simulink model "test_newfft"  (Simulink 6.2)
settings: Solver=ode45  StartTime=0.0  StopTime=100  RelTol=1e-3
libraries: xbsIndex_r3 x265, simulink x1
(part 2 of 4)

== system test_newfft/r2_dit_fft/r2_dit_stage_1 ==
  a_in : Inport  Port=1  LatchInput=off
  b_in : Inport  Port=2  LatchInput=off
  sync_in : Inport  Port=3  LatchInput=off
  biplex_commutator : Subsystem  mask(Biplex Commutator){log2_size=4, n_bits=8, use_bram=off}
      mask prompts: log2_size "Log2 Block Size"; n_bits "Bit Width"; use_bram "Use BRAM"
      mask help: The biplex commutator commutes the first half of the BloBhi input "block" with the last half of the AloAhi input "block". A "block" is 2^log2_size consecutive samples (i.e. always a power of 2). sync_in precedes the first data input sample by one clock cycle. Overall latency from sync_in to sync_out is 2^(log2_size-1)+1.
      settings: AttributesFormatString=|
      | size = 16
      | delay slr
      mask Help:
      | <pre>
      | Description::
      | 
      | The biplex commutator commutes the first half of the BloBhi input "block"  with the last half
      | of the AloAhi input "block".  A "block" is 2^log2_size consecutive samples (i.e. always a
      | power of 2).
      | 
      | sync_in precedes the first data input sample by one clock cycle.
      | sync_out precedes the corresponding output sample by one clock cycle.
      | Overall latency from sync_in to sync_out is 2^(N-1)+1.
      | 
      | Mask Parameters::
      | 
      | Log 2 Block Size (log2_size): The base-2 logarithm of the length of one complete input block.
      | This MUST be an integer because the current implementation requires that
      | the input block size MUST be a power of 2.  (aka "N")
      | 
      | Bit Width (n_bits): Specifies the width of the real/imaginary components.
      | Width of each component is assumed equal.
      | 
      | Use BRAM (use_bram): Check this checkbox to implement the internal delays using BRAM.
      | If unchecked, the internal delays will be implemented using SLR16 elements.
      | </pre>
  r2_butterfly : Subsystem  mask(Radix-2 Butterfly){n_bits=8, shift=0, quantization=Truncate, add_latency=1}
      mask prompts: n_bits "Bit Width In"; shift "Shift Bits"; add_latency "Adder Latency"
      mask help: The radix-2 butterfly produces a+b and a-b outputs for a and b inputs.
      settings: AttributesFormatString=shift 0
      mask Help:
      | <pre>
      | Description::
      | 
      | The radix-2 butterfly produces a+b and a-b outputs for a and b inputs.
      | The outputs are one bit wider than the inputs.
      | The output precision (i.e. the number of fractional bits) stays the same.
      | 
      | Mask Parameters::
      | 
      | Bit Width In (n_bits): Specifies the width of the real/imaginary components.
      | Width of each component is assumed equal.
      | 
      | Shift Bits (shift): Specifies how many bits to shift (down) by.  A positive value causes
      | the specified number of least significant bits to be dropped.  Usually zero or positive values
      | are used to permit or limit bit growth, but negative values can be used to induce bit growth.
      | 
      | Quantization (quantization): Specifies quantization handling (when shift bits > 0).
      | 
      | Adder Latency (add_latency): Latency to use for the underlying real adders.
      | </pre>
      mask StyleString: edit,edit,popup(Truncate|Round  (unbiased: +/- Inf)|Round  (unbiased: Even Values)),edit
  r2_twiddle : Subsystem
      mask Type: Radix-2 Stage-1 Twiddle Stage
      mask Description: A stage-1 twiddle stage for radix-2 Fast Fourier Transforms. Since there are no twiddles in stage 1 of an FFT, this is just a dummy placeholder block that passes its inputs through to its outputs.    Since it is a no-op, its use is completely optional.
      mask Help:
      | <pre>
      | Description::
      | 
      | A stage-1 twiddle stage for radix-2 Fast Fourier Transforms.
      | 
      | Since there are no twiddles in stage 1 of an FFT, this is just a dummy placeholder
      | block that passes its inputs through to its outputs.
      | 
      | Since it is a no-op, its use is completely optional.
      | 
      | Note that stages are counted from 1 to n_stages for DIT (i.e. cur_stage==1 for the first stage)
      | and n_stages to 1for DIF (i.e. cur_stage==1 for the last stage).  Therefore, this block, if used,
      | should be the first twiddle stage of a DIT FFT or the last twiddle stage of a DIF FFT.
      | 
      | Mask Parameters::
      | 
      | (N/A)
  a_out : Outport
  b_out : Outport  Port=2
  sync_out : Outport  Port=3
  wires:
  r2_butterfly/3(sync_out) -> sync_out/1
  r2_butterfly/2(a-b) -> b_out/1
  r2_butterfly/1(a+b) -> a_out/1
  sync_in/1 -> biplex_commutator/3(sync_in)
  b_in/1 -> biplex_commutator/2(BloBhi)
  a_in/1 -> biplex_commutator/1(AloAhi)
  biplex_commutator/3(sync_out) -> r2_twiddle/3(sync_in)
  biplex_commutator/2(AhiBhi) -> r2_twiddle/2(b_in)
  biplex_commutator/1(AloBlo) -> r2_twiddle/1(a_in)
  r2_twiddle/1(a_out) -> r2_butterfly/1(a)
  r2_twiddle/2(b_out) -> r2_butterfly/2(b)
  r2_twiddle/3(sync_out) -> r2_butterfly/3(sync_in)

== system test_newfft/r2_dit_fft/r2_dit_stage_2 ==
  a_in : Inport  Port=1  LatchInput=off
  b_in : Inport  Port=2  LatchInput=off
  sync_in : Inport  Port=3  LatchInput=off
  biplex_commutator : Subsystem  mask(Biplex Commutator){log2_size=3, n_bits=9, use_bram=off}
      mask prompts: log2_size "Log2 Block Size"; n_bits "Bit Width"; use_bram "Use BRAM"
      mask help: The biplex commutator commutes the first half of the BloBhi input "block" with the last half of the AloAhi input "block". A "block" is 2^log2_size consecutive samples (i.e. always a power of 2). sync_in precedes the first data input sample by one clock cycle. Overall latency from sync_in to sync_out is 2^(log2_size-1)+1.
      settings: AttributesFormatString=|
      | size = 8
      | delay slr
      mask Help:
      | <pre>
      | Description::
      | 
      | The biplex commutator commutes the first half of the BloBhi input "block"  with the last half
      | of the AloAhi input "block".  A "block" is 2^log2_size consecutive samples (i.e. always a
      | power of 2).
      | 
      | sync_in precedes the first data input sample by one clock cycle.
      | sync_out precedes the corresponding output sample by one clock cycle.
      | Overall latency from sync_in to sync_out is 2^(N-1)+1.
      | 
      | Mask Parameters::
      | 
      | Log 2 Block Size (log2_size): The base-2 logarithm of the length of one complete input block.
      | This MUST be an integer because the current implementation requires that
      | the input block size MUST be a power of 2.  (aka "N")
      | 
      | Bit Width (n_bits): Specifies the width of the real/imaginary components.
      | Width of each component is assumed equal.
      | 
      | Use BRAM (use_bram): Check this checkbox to implement the internal delays using BRAM.
      | If unchecked, the internal delays will be implemented using SLR16 elements.
      | </pre>
  r2_butterfly : Subsystem  mask(Radix-2 Butterfly with optional -j twiddle (DIT, twiddle before butterfly)){n_bits=9, shift=0, quantization=Truncate, add_latency=1}
      mask prompts: n_bits "Bit Width In"; shift "Shift Bits"; add_latency "Adder Latency"
      mask help: The radix-2 butterfly produces a+b and a-b outputs for a and b inputs. This variation efficiently includes an optional -j twiddle factor that can be applied before the butterfly (suitable for use in stage two of a DIT FFT).
      settings: AttributesFormatString=shift 0
      mask Help:
      | <pre>
      | Description::
      | 
      | The radix-2 butterfly produces a+b and a-b outputs for a and b inputs.
      | This variation efficiently includes an optional -j twiddle factor that can be
      | applied before the butterfly (suitable for use in stage two of a DIT FFT).
      | 
      | The -j twiddle factor is applied to tbe b input when tw_en is high,
      | thus producing a-jb on the a+b output and a+jb on the a-b output.
      | 
      | The outputs are one bit wider than the inputs.
      | The output precision (i.e. the number of fractional bits) stays the same.
      | 
      | Mask Parameters::
      | 
      | Bit Width In (n_bits): Specifies the width of the real/imaginary components.
      | Width of each component is assumed equal.
      | 
      | Shift Bits (shift): Specifies how many bits to shift (down) by.  A positive value causes
      | the specified number of least significant bits to be dropped.  Usually zero or positive values
      | are used to permit or limit bit growth, but negative values can be used to induce bit growth.
      | 
      | Quantization (quantization): Specifies quantization handling (when shift bits > 0).
      | 
      | Adder Latency (add_latency): Latency to use for the underlying real adders.
      | </pre>
      mask StyleString: edit,edit,popup(Truncate|Round  (unbiased: +/- Inf)|Round  (unbiased: Even Values)),edit
  r2_twiddle : Subsystem  mask(Radix-2 DIT Stage-2 Twiddle Stage){n_stages=4}
      mask prompts: n_stages "Total Stages"
      mask help: A stage-2 twiddle stage for radix-2 Decimation in Time Fast Fourier Transforms. The FFT is assumed to have inputs in normal order and outputs in bit-reversed order. This block must be used in conjuction with an r2_butterfly_dit_j_opt block (or equivalent) which has an optional -j twiddle factor built in.
      mask Help:
      | <pre>
      | Description::
      | 
      | A stage-2 twiddle stage for radix-2 Decimation in Time Fast Fourier Transforms.
      | 
      | The FFT is assumed to have inputs in normal order and outputs in bit-reversed order.
      | 
      | This block must be used in conjuction with an r2_butterfly_dit_j_opt block (or equivalent)
      | which has an optional -j twiddle factor built in.  This block does no twidlling at all; it just provides
      | a tw_en output for use with an r2_butterfly_dit_j_opt block (or equivalent).
      | 
      | Mask Parameters::
      | 
      | Total Stages (n_stages):  The number of total stages in the FFT.
      | The FFT will have 2^n_stages points.
  a_out : Outport
  b_out : Outport  Port=2
  sync_out : Outport  Port=3
  wires:
  r2_butterfly/3(sync_out) -> sync_out/1
  r2_butterfly/2(a-b) -> b_out/1
  r2_butterfly/1(a+b) -> a_out/1
  sync_in/1 -> biplex_commutator/3(sync_in)
  b_in/1 -> biplex_commutator/2(BloBhi)
  a_in/1 -> biplex_commutator/1(AloAhi)
  biplex_commutator/3(sync_out) -> r2_twiddle/3(sync_in)
  biplex_commutator/2(AhiBhi) -> r2_twiddle/2(b_in)
  biplex_commutator/1(AloBlo) -> r2_twiddle/1(a_in)
  r2_twiddle/1(a_out) -> r2_butterfly/1(a)
  r2_twiddle/2(b_out) -> r2_butterfly/2(b)
  r2_twiddle/3(sync_out) -> r2_butterfly/3(sync_in)
  r2_twiddle/4(tw_en) -> r2_butterfly/4(tw_en)

== system test_newfft/r2_dit_fft/r2_dit_stage_3 ==
  a_in : Inport  Port=1  LatchInput=off
  b_in : Inport  Port=2  LatchInput=off
  sync_in : Inport  Port=3  LatchInput=off
  biplex_commutator : Subsystem  mask(Biplex Commutator){log2_size=2, n_bits=10, use_bram=off}
      mask prompts: log2_size "Log2 Block Size"; n_bits "Bit Width"; use_bram "Use BRAM"
      mask help: The biplex commutator commutes the first half of the BloBhi input "block" with the last half of the AloAhi input "block". A "block" is 2^log2_size consecutive samples (i.e. always a power of 2). sync_in precedes the first data input sample by one clock cycle. Overall latency from sync_in to sync_out is 2^(log2_size-1)+1.
      settings: AttributesFormatString=|
      | size = 4
      | delay slr
      mask Help:
      | <pre>
      | Description::
      | 
      | The biplex commutator commutes the first half of the BloBhi input "block"  with the last half
      | of the AloAhi input "block".  A "block" is 2^log2_size consecutive samples (i.e. always a
      | power of 2).
      | 
      | sync_in precedes the first data input sample by one clock cycle.
      | sync_out precedes the corresponding output sample by one clock cycle.
      | Overall latency from sync_in to sync_out is 2^(N-1)+1.
      | 
      | Mask Parameters::
      | 
      | Log 2 Block Size (log2_size): The base-2 logarithm of the length of one complete input block.
      | This MUST be an integer because the current implementation requires that
      | the input block size MUST be a power of 2.  (aka "N")
      | 
      | Bit Width (n_bits): Specifies the width of the real/imaginary components.
      | Width of each component is assumed equal.
      | 
      | Use BRAM (use_bram): Check this checkbox to implement the internal delays using BRAM.
      | If unchecked, the internal delays will be implemented using SLR16 elements.
      | </pre>
  r2_butterfly : Subsystem  mask(Radix-2 Butterfly){n_bits=10, shift=0, quantization=Truncate, add_latency=1}
      mask prompts: n_bits "Bit Width In"; shift "Shift Bits"; add_latency "Adder Latency"
      mask help: The radix-2 butterfly produces a+b and a-b outputs for a and b inputs.
      settings: AttributesFormatString=shift 0
      mask Help:
      | <pre>
      | Description::
      | 
      | The radix-2 butterfly produces a+b and a-b outputs for a and b inputs.
      | The outputs are one bit wider than the inputs.
      | The output precision (i.e. the number of fractional bits) stays the same.
      | 
      | Mask Parameters::
      | 
      | Bit Width In (n_bits): Specifies the width of the real/imaginary components.
      | Width of each component is assumed equal.
      | 
      | Shift Bits (shift): Specifies how many bits to shift (down) by.  A positive value causes
      | the specified number of least significant bits to be dropped.  Usually zero or positive values
      | are used to permit or limit bit growth, but negative values can be used to induce bit growth.
      | 
      | Quantization (quantization): Specifies quantization handling (when shift bits > 0).
      | 
      | Adder Latency (add_latency): Latency to use for the underlying real adders.
      | </pre>
      mask StyleString: edit,edit,popup(Truncate|Round  (unbiased: +/- Inf)|Round  (unbiased: Even Values)),edit
  r2_twiddle : Subsystem  mask(Radix-2 General Twiddle Stage){n_stages=4, cur_stage=3, decimation=Time, n_bits=10, bin_pt=7, n_bits_w=9, use_bram=off, mult_latency=3, add_latency=1}
      mask prompts: n_stages "Total Stages"; cur_stage "Current Stage"; decimation "Decimation Mode"; n_bits "Number of Bits In/Out"; bin_pt "Binary Point In/Out"; n_bits_w "Twiddle Coefficient Bitwidth"; use_bram "Use BRAM For Twiddle Coefficients"; mult_latency "Multiplier Latency"; add_latency "Adder Latency"
      mask help: A general twiddle stage for radix-2 Fast Fourier Transforms. Can be used in Decimation in Time (i.e. twiddles before butterflies) or Decimation in Frequency (i.e. twiddles after butterflies) FFTs. Regardless of the decimation mode, the FFT is assumed to have inputs in normal order and outputs in bit-reversed order.
      settings: AttributesFormatString=4 twiddles in dist
      mask Help:
      | <pre>
      | Description::
      | 
      | A general twiddle stage for radix-2 Fast Fourier Transforms.
      | 
      | Can be used in  Decimation in Time (i.e. twiddles before butterflies) or Decimation in Frequency
      | (i.e. twiddles after butterflies) FFTs.  Regardless of the decimation mode, the FFT is assumed
      | to have inputs in normal order and outputs in bit-reversed order.
      | 
      | Input a_in is passed through unchanged to a_out, while input b is passed through to bw after
      | being "twiddled".  Since twiddling is effectively multiplication by a complex number with unity
      | magnitude, the bit respresentation of bw is the same as b (i.e. twiddling does not cause bit
      | growth).  Input a_in is assumed to have the same bit width as b.  Thus, a_in, a_out, b, and
      | bw all have the same bit representation.
      | 
      | Mask Parameters::
      | 
      | Total Stages (n_stages):  The number of total stages in the FFT.
      | The FFT will have 2^n_stages points.
      | 
      | Current Stage (cur_stage):  The number of the current stage for which this block should
      | generate twiddle coefficients.  Valid values are 3 through n_stages, inclusive.  Note that
      | stages are counted from 1 to n_stages for DIT (i.e. cur_stage==1 for the first stage) and
      | n_stages to 1 for DIF (i.e. cur_stage==1 for the last stage).
      | 
      | Decimation Mode (decimation): The decimation mode of the FFT.
      | 
      | Number of Bits In/Out (n_bits): Specifies the width of the real/imaginary
      | components of ports a_in, b, a_out, bw.  Assumed equal for both components.
      | 
      | Binary Point In/Out (bin_pt): Specifies the binary point position of the real/imaginary
      | components of ports a_in, b, a_out, bw.  Assumed equal for both components.
      | 
      | Twiddle Coefficient Bitwidth (n_bits_w): Specifies the width of the real/imaginary
      | components of the twiddle coefficients.  Assumed equal for both components.
      | 
      | Use BRAM for Twiddle Coefficients (use_bram): Check this checkbox to store twiddle
      | coefficients in BRAM.  If unchecked, the twiddle coefficients will be sored in distributed
      | memory (i.e. slices).
      | 
      | Multiplier Latency (mult_latency): Latency to use for the underlying real multipliers.
      | 
      | Adder Latency (add_latency): Latency to use for the underlying real adders.
      mask StyleString: edit,edit,popup(Time|Frequency),edit,edit,edit,checkbox,edit,edit
  a_out : Outport
  b_out : Outport  Port=2
  sync_out : Outport  Port=3
  wires:
  r2_butterfly/3(sync_out) -> sync_out/1
  r2_butterfly/2(a-b) -> b_out/1
  r2_butterfly/1(a+b) -> a_out/1
  sync_in/1 -> biplex_commutator/3(sync_in)
  b_in/1 -> biplex_commutator/2(BloBhi)
  a_in/1 -> biplex_commutator/1(AloAhi)
  biplex_commutator/3(sync_out) -> r2_twiddle/3(sync_in)
  biplex_commutator/2(AhiBhi) -> r2_twiddle/2(b)
  biplex_commutator/1(AloBlo) -> r2_twiddle/1(a_in)
  r2_twiddle/1(a_out) -> r2_butterfly/1(a)
  r2_twiddle/2(bw) -> r2_butterfly/2(b)
  r2_twiddle/3(sync_out) -> r2_butterfly/3(sync_in)

== system test_newfft/r2_dit_fft/r2_dit_stage_4 ==
  a_in : Inport  Port=1  LatchInput=off
  b_in : Inport  Port=2  LatchInput=off
  sync_in : Inport  Port=3  LatchInput=off
  biplex_commutator : Subsystem  mask(Biplex Commutator){log2_size=1, n_bits=11, use_bram=off}
      mask prompts: log2_size "Log2 Block Size"; n_bits "Bit Width"; use_bram "Use BRAM"
      mask help: The biplex commutator commutes the first half of the BloBhi input "block" with the last half of the AloAhi input "block". A "block" is 2^log2_size consecutive samples (i.e. always a power of 2). sync_in precedes the first data input sample by one clock cycle. Overall latency from sync_in to sync_out is 2^(log2_size-1)+1.
      settings: AttributesFormatString=|
      | size = 2
      | delay slr
      mask Help:
      | <pre>
      | Description::
      | 
      | The biplex commutator commutes the first half of the BloBhi input "block"  with the last half
      | of the AloAhi input "block".  A "block" is 2^log2_size consecutive samples (i.e. always a
      | power of 2).
      | 
      | sync_in precedes the first data input sample by one clock cycle.
      | sync_out precedes the corresponding output sample by one clock cycle.
      | Overall latency from sync_in to sync_out is 2^(N-1)+1.
      | 
      | Mask Parameters::
      | 
      | Log 2 Block Size (log2_size): The base-2 logarithm of the length of one complete input block.
      | This MUST be an integer because the current implementation requires that
      | the input block size MUST be a power of 2.  (aka "N")
      | 
      | Bit Width (n_bits): Specifies the width of the real/imaginary components.
      | Width of each component is assumed equal.
      | 
      | Use BRAM (use_bram): Check this checkbox to implement the internal delays using BRAM.
      | If unchecked, the internal delays will be implemented using SLR16 elements.
      | </pre>
  r2_butterfly : Subsystem  mask(Radix-2 Butterfly){n_bits=11, shift=0, quantization=Truncate, add_latency=1}
      mask prompts: n_bits "Bit Width In"; shift "Shift Bits"; add_latency "Adder Latency"
      mask help: The radix-2 butterfly produces a+b and a-b outputs for a and b inputs.
      settings: AttributesFormatString=shift 0
      mask Help:
      | <pre>
      | Description::
      | 
      | The radix-2 butterfly produces a+b and a-b outputs for a and b inputs.
      | The outputs are one bit wider than the inputs.
      | The output precision (i.e. the number of fractional bits) stays the same.
      | 
      | Mask Parameters::
      | 
      | Bit Width In (n_bits): Specifies the width of the real/imaginary components.
      | Width of each component is assumed equal.
      | 
      | Shift Bits (shift): Specifies how many bits to shift (down) by.  A positive value causes
      | the specified number of least significant bits to be dropped.  Usually zero or positive values
      | are used to permit or limit bit growth, but negative values can be used to induce bit growth.
      | 
      | Quantization (quantization): Specifies quantization handling (when shift bits > 0).
      | 
      | Adder Latency (add_latency): Latency to use for the underlying real adders.
      | </pre>
      mask StyleString: edit,edit,popup(Truncate|Round  (unbiased: +/- Inf)|Round  (unbiased: Even Values)),edit
  r2_twiddle : Subsystem  mask(Radix-2 General Twiddle Stage){n_stages=4, cur_stage=4, decimation=Time, n_bits=11, bin_pt=7, n_bits_w=9, use_bram=off, mult_latency=3, add_latency=1}
      mask prompts: n_stages "Total Stages"; cur_stage "Current Stage"; decimation "Decimation Mode"; n_bits "Number of Bits In/Out"; bin_pt "Binary Point In/Out"; n_bits_w "Twiddle Coefficient Bitwidth"; use_bram "Use BRAM For Twiddle Coefficients"; mult_latency "Multiplier Latency"; add_latency "Adder Latency"
      mask help: A general twiddle stage for radix-2 Fast Fourier Transforms. Can be used in Decimation in Time (i.e. twiddles before butterflies) or Decimation in Frequency (i.e. twiddles after butterflies) FFTs. Regardless of the decimation mode, the FFT is assumed to have inputs in normal order and outputs in bit-reversed order.
      settings: AttributesFormatString=8 twiddles in dist
      mask Help:
      | <pre>
      | Description::
      | 
      | A general twiddle stage for radix-2 Fast Fourier Transforms.
      | 
      | Can be used in  Decimation in Time (i.e. twiddles before butterflies) or Decimation in Frequency
      | (i.e. twiddles after butterflies) FFTs.  Regardless of the decimation mode, the FFT is assumed
      | to have inputs in normal order and outputs in bit-reversed order.
      | 
      | Input a_in is passed through unchanged to a_out, while input b is passed through to bw after
      | being "twiddled".  Since twiddling is effectively multiplication by a complex number with unity
      | magnitude, the bit respresentation of bw is the same as b (i.e. twiddling does not cause bit
      | growth).  Input a_in is assumed to have the same bit width as b.  Thus, a_in, a_out, b, and
      | bw all have the same bit representation.
      | 
      | Mask Parameters::
      | 
      | Total Stages (n_stages):  The number of total stages in the FFT.
      | The FFT will have 2^n_stages points.
      | 
      | Current Stage (cur_stage):  The number of the current stage for which this block should
      | generate twiddle coefficients.  Valid values are 3 through n_stages, inclusive.  Note that
      | stages are counted from 1 to n_stages for DIT (i.e. cur_stage==1 for the first stage) and
      | n_stages to 1 for DIF (i.e. cur_stage==1 for the last stage).
      | 
      | Decimation Mode (decimation): The decimation mode of the FFT.
      | 
      | Number of Bits In/Out (n_bits): Specifies the width of the real/imaginary
      | components of ports a_in, b, a_out, bw.  Assumed equal for both components.
      | 
      | Binary Point In/Out (bin_pt): Specifies the binary point position of the real/imaginary
      | components of ports a_in, b, a_out, bw.  Assumed equal for both components.
      | 
      | Twiddle Coefficient Bitwidth (n_bits_w): Specifies the width of the real/imaginary
      | components of the twiddle coefficients.  Assumed equal for both components.
      | 
      | Use BRAM for Twiddle Coefficients (use_bram): Check this checkbox to store twiddle
      | coefficients in BRAM.  If unchecked, the twiddle coefficients will be sored in distributed
      | memory (i.e. slices).
      | 
      | Multiplier Latency (mult_latency): Latency to use for the underlying real multipliers.
      | 
      | Adder Latency (add_latency): Latency to use for the underlying real adders.
      mask StyleString: edit,edit,popup(Time|Frequency),edit,edit,edit,checkbox,edit,edit
  a_out : Outport
  b_out : Outport  Port=2
  sync_out : Outport  Port=3
  wires:
  r2_butterfly/3(sync_out) -> sync_out/1
  r2_butterfly/2(a-b) -> b_out/1
  r2_butterfly/1(a+b) -> a_out/1
  sync_in/1 -> biplex_commutator/3(sync_in)
  b_in/1 -> biplex_commutator/2(BloBhi)
  a_in/1 -> biplex_commutator/1(AloAhi)
  biplex_commutator/3(sync_out) -> r2_twiddle/3(sync_in)
  biplex_commutator/2(AhiBhi) -> r2_twiddle/2(b)
  biplex_commutator/1(AloBlo) -> r2_twiddle/1(a_in)
  r2_twiddle/1(a_out) -> r2_butterfly/1(a)
  r2_twiddle/2(bw) -> r2_butterfly/2(b)
  r2_twiddle/3(sync_out) -> r2_butterfly/3(sync_in)

== system test_newfft/r2_dit_fft/biplex_bitrev/bit_reverse ==
  in : Inport  Port=1  LatchInput=off
  bit0 : xbsIndex_r3/Slice  mode=Lower Bit Location + Width  nbits=1  bit1=0  base1=MSB of Input  bit0=0  base0=LSB of Input  boolean_output=off  explicit_period=off  period=1  dbl_ovrd=off
  bit1 : xbsIndex_r3/Slice  mode=Lower Bit Location + Width  nbits=1  bit1=0  base1=MSB of Input  bit0=1  base0=LSB of Input  boolean_output=off  explicit_period=off  period=1  dbl_ovrd=off
  bit2 : xbsIndex_r3/Slice  mode=Lower Bit Location + Width  nbits=1  bit1=0  base1=MSB of Input  bit0=2  base0=LSB of Input  boolean_output=off  explicit_period=off  period=1  dbl_ovrd=off
  concat : xbsIndex_r3/Concat  num_inputs=3  explicit_period=off  period=1  dbl_ovrd=off
  out : Outport
  wires:
  in/1 -> bit2/1, bit1/1, bit0/1
  bit2/1 -> concat/3
  bit1/1 -> concat/2
  bit0/1 -> concat/1
  concat/1 -> out/1

== system test_newfft/r2_dit_fft/biplex_bitrev/c_to_ri ==
  c : Inport  Port=1  LatchInput=off
  force_im : xbsIndex_r3/Reinterpret  force_arith_type=on  arith_type="Signed  (2's comp)"  force_bin_pt=on  bin_pt=0  force_valid=on
  force_re : xbsIndex_r3/Reinterpret  force_arith_type=on  arith_type="Signed  (2's comp)"  force_bin_pt=on  bin_pt=0  force_valid=on
  slice_im : xbsIndex_r3/Slice  mode=Lower Bit Location + Width  nbits=12  bit1=0  base1=MSB of Input  bit0=0  base0=LSB of Input  boolean_output=off  explicit_period=off  period=1  dbl_ovrd=off
  slice_re : xbsIndex_r3/Slice  mode=Upper Bit Location + Width  nbits=12  bit1=0  base1=MSB of Input  bit0=0  base0=LSB of Input  boolean_output=off  explicit_period=off  period=1  dbl_ovrd=off
  re : Outport
  im : Outport  Port=2
  wires:
  slice_re/1 -> force_re/1
  slice_im/1 -> force_im/1
  force_re/1 -> re/1
  force_im/1 -> im/1
  c/1 -> slice_re/1, slice_im/1

== system test_newfft/r2_dit_fft/biplex_bitrev/c_to_ri1 ==
  c : Inport  Port=1  LatchInput=off
  force_im : xbsIndex_r3/Reinterpret  force_arith_type=on  arith_type="Signed  (2's comp)"  force_bin_pt=on  bin_pt=0  force_valid=on
  force_re : xbsIndex_r3/Reinterpret  force_arith_type=on  arith_type="Signed  (2's comp)"  force_bin_pt=on  bin_pt=0  force_valid=on
  slice_im : xbsIndex_r3/Slice  mode=Lower Bit Location + Width  nbits=12  bit1=0  base1=MSB of Input  bit0=0  base0=LSB of Input  boolean_output=off  explicit_period=off  period=1  dbl_ovrd=off
  slice_re : xbsIndex_r3/Slice  mode=Upper Bit Location + Width  nbits=12  bit1=0  base1=MSB of Input  bit0=0  base0=LSB of Input  boolean_output=off  explicit_period=off  period=1  dbl_ovrd=off
  re : Outport
  im : Outport  Port=2
  wires:
  slice_re/1 -> force_re/1
  slice_im/1 -> force_im/1
  force_re/1 -> re/1
  force_im/1 -> im/1
  c/1 -> slice_re/1, slice_im/1

== system test_newfft/r2_dit_fft/biplex_bitrev/ri_to_c ==
  re : Inport  Port=1  LatchInput=off
  im : Inport  Port=2  LatchInput=off
  concat : xbsIndex_r3/Concat  num_inputs=2  explicit_period=off  period=1  dbl_ovrd=off
  force_im : xbsIndex_r3/Reinterpret  force_arith_type=on  arith_type=Unsigned  force_bin_pt=on  bin_pt=0  force_valid=on
  force_re : xbsIndex_r3/Reinterpret  force_arith_type=on  arith_type=Unsigned  force_bin_pt=on  bin_pt=0  force_valid=on
  c : Outport
  wires:
  force_re/1 -> concat/1
  force_im/1 -> concat/2
  re/1 -> force_re/1
  concat/1 -> c/1
  im/1 -> force_im/1

== system test_newfft/r2_dit_fft/biplex_bitrev/ri_to_c1 ==
  re : Inport  Port=1  LatchInput=off
  im : Inport  Port=2  LatchInput=off
  concat : xbsIndex_r3/Concat  num_inputs=2  explicit_period=off  period=1  dbl_ovrd=off
  force_im : xbsIndex_r3/Reinterpret  force_arith_type=on  arith_type=Unsigned  force_bin_pt=on  bin_pt=0  force_valid=on
  force_re : xbsIndex_r3/Reinterpret  force_arith_type=on  arith_type=Unsigned  force_bin_pt=on  bin_pt=0  force_valid=on
  c : Outport
  wires:
  force_re/1 -> concat/1
  force_im/1 -> concat/2
  re/1 -> force_re/1
  concat/1 -> c/1
  im/1 -> force_im/1

== system test_newfft/r2_dit_fft/biplex_commutator/delay_b ==
  in : Inport  Port=1  LatchInput=off
  slr : xbsIndex_r3/Delay  latency=8  reg_retiming=off  explicit_period=off  period=1  en=off  accept_only_valid=off  init_zero=on  dbl_ovrd=off  show_param=off
      settings: xl_area=[0, 0, 0, 0, 0, 0, 0]
  out : Outport
  wires:
  slr/1 -> out/1
  in/1 -> slr/1

== system test_newfft/r2_dit_fft/biplex_commutator/delay_lo ==
  in : Inport  Port=1  LatchInput=off
  slr : xbsIndex_r3/Delay  latency=8  reg_retiming=off  explicit_period=off  period=1  en=off  accept_only_valid=off  init_zero=on  dbl_ovrd=off  show_param=off
      settings: xl_area=[0, 0, 0, 0, 0, 0, 0]
  out : Outport
  wires:
  slr/1 -> out/1
  in/1 -> slr/1

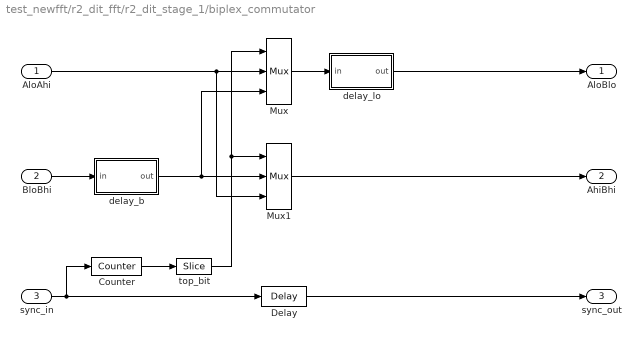
== system test_newfft/r2_dit_fft/r2_dit_stage_1/biplex_commutator ==
  AloAhi : Inport  Port=1  LatchInput=off
  BloBhi : Inport  Port=2  LatchInput=off
  sync_in : Inport  Port=3  LatchInput=off
  Counter : xbsIndex_r3/Counter  cnt_type=Free Running  n_bits=4  bin_pt=0  arith_type=Unsigned  start_count=0  cnt_to=Inf  cnt_by_val=1  operation=Up  explicit_period=off  period=1  load_pin=off  rst=on  en=off  dbl_ovrd=off  show_param=off  use_rpm=on  gen_core=off
      settings: xl_area=[0, 0, 0, 0, 0, 0, 0]
  Delay : xbsIndex_r3/Delay  latency=9  reg_retiming=off  explicit_period=off  period=1  en=off  accept_only_valid=off  init_zero=on  dbl_ovrd=off  show_param=off
      settings: xl_area=[0, 0, 0, 0, 0, 0, 0]
  Mux : xbsIndex_r3/Mux  inputs=2  precision=Full  arith_type="Signed  (2's comp)"  n_bits=8  bin_pt=2  quantization=Truncate  overflow=Wrap  latency=1  explicit_period=off  period=1  en=off  dbl_ovrd=off  show_param=off  mux_type=off  use_rpm=off  gen_core=off
      settings: xl_area=[0, 0, 0, 0, 0, 0, 0]
  Mux1 : xbsIndex_r3/Mux  inputs=2  precision=Full  arith_type="Signed  (2's comp)"  n_bits=8  bin_pt=2  quantization=Truncate  overflow=Wrap  latency=1  explicit_period=off  period=1  en=off  dbl_ovrd=off  show_param=on  mux_type=off  use_rpm=off  gen_core=off
      settings: xl_area=[0, 0, 0, 0, 0, 0, 0]
  delay_b : Subsystem  mask(SLR16 Delay){delay_depth=8}
      mask prompts: delay_depth "Delay Depth"
      mask help: A delay block that uses SLR16 elements for its storage.
      settings: AttributesFormatString=slr depth = 8
      mask Help:
      | <pre>
      | Description::
      | 
      | A delay block that uses SLR16 elements for its storage.
      | 
      | Mask Parameters::
      | 
      | Delay Depth (delay_depth): The length of the delay.
      | </pre>
  delay_lo : Subsystem  mask(SLR16 Delay){delay_depth=8}
      mask prompts: delay_depth "Delay Depth"
      mask help: A delay block that uses SLR16 elements for its storage.
      settings: AttributesFormatString=slr depth = 8
      mask Help:
      | <pre>
      | Description::
      | 
      | A delay block that uses SLR16 elements for its storage.
      | 
      | Mask Parameters::
      | 
      | Delay Depth (delay_depth): The length of the delay.
      | </pre>
  top_bit : xbsIndex_r3/Slice  mode=Upper Bit Location + Width  nbits=1  bit1=0  base1=MSB of Input  bit0=0  base0=LSB of Input  boolean_output=off  explicit_period=off  period=1  dbl_ovrd=off
  AloBlo : Outport
  AhiBhi : Outport  Port=2
  sync_out : Outport  Port=3
  wires:
  Delay/1 -> sync_out/1
  delay_lo/1(out) -> AloBlo/1
  Mux/1 -> delay_lo/1(in)
  delay_b/1(out) -> Mux/3, Mux1/2
  BloBhi/1 -> delay_b/1(in)
  Mux1/1 -> AhiBhi/1
  AloAhi/1 -> Mux1/3, Mux/2
  top_bit/1 -> Mux/1, Mux1/1
  Counter/1 -> top_bit/1
  sync_in/1 -> Delay/1, Counter/1

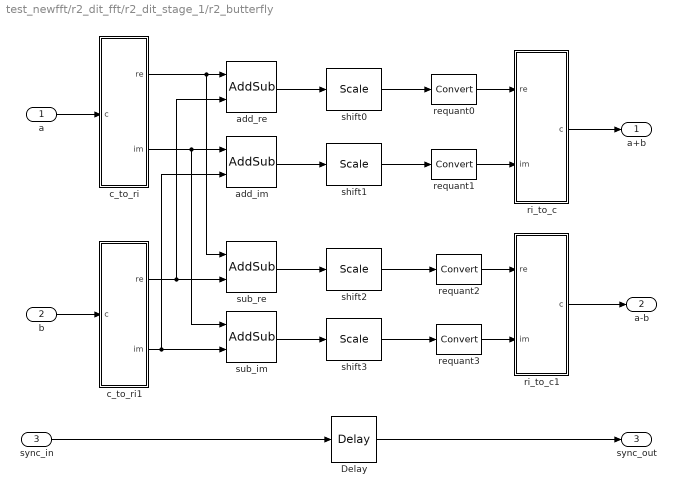
== system test_newfft/r2_dit_fft/r2_dit_stage_1/r2_butterfly ==
  a : Inport  Port=1  LatchInput=off
  b : Inport  Port=2  LatchInput=off
  sync_in : Inport  Port=3  LatchInput=off
  Delay : xbsIndex_r3/Delay  latency=1  reg_retiming=off  explicit_period=off  period=1  en=off  accept_only_valid=off  init_zero=on  dbl_ovrd=off  show_param=off
      settings: xl_area=[0, 0, 0, 0, 0, 0, 0]
  add_im : xbsIndex_r3/AddSub  mode=Addition  precision=Full  arith_type=Unsigned  n_bits=8  bin_pt=2  quantization=Truncate  overflow=Wrap  latency=1  explicit_period=off  period=1  use_carryin=off  use_carryout=off  en=off  dbl_ovrd=off  show_param=on  use_core=on  pipeline=on  use_rpm=on  gen_core=off
      settings: xl_area=[0, 0, 0, 0, 0, 0, 0]
  add_re : xbsIndex_r3/AddSub  mode=Addition  precision=Full  arith_type=Unsigned  n_bits=8  bin_pt=2  quantization=Truncate  overflow=Wrap  latency=1  explicit_period=off  period=1  use_carryin=off  use_carryout=off  en=off  dbl_ovrd=off  show_param=on  use_core=on  pipeline=on  use_rpm=on  gen_core=off
      settings: xl_area=[0, 0, 0, 0, 0, 0, 0]
  c_to_ri : Subsystem  mask(Complex to Real-Imag){n_bits=8, bin_pt=0}
      mask prompts: n_bits "Bit Width"; bin_pt "Binary Point"
      mask help: Outputs real and imaginary components of a complex input.
      settings: AttributesFormatString=8_0 r/i
      mask Help:
      | <pre>
      | Description::
      | 
      | Outputs real and imaginary components of a complex input.
      | Useful for simplifying interconnects.
      | See also: Real-Imag to Complex (ri_to_c)
      | 
      | Mask Parameters::
      | 
      | Bit Width (n_bits): Specifies the width of the real/imaginary components.
      | Assumed equal for both components.
      | 
      | Binary Point (bin_pt): Specifies the binary point location in the real/imaginary components.
      | Assumed equal for both components.
      | </pre>
  c_to_ri1 : Subsystem  mask(Complex to Real-Imag){n_bits=8, bin_pt=0}
      mask prompts: n_bits "Bit Width"; bin_pt "Binary Point"
      mask help: Outputs real and imaginary components of a complex input.
      settings: AttributesFormatString=8_0 r/i
      mask Help:
      | <pre>
      | Description::
      | 
      | Outputs real and imaginary components of a complex input.
      | Useful for simplifying interconnects.
      | See also: Real-Imag to Complex (ri_to_c)
      | 
      | Mask Parameters::
      | 
      | Bit Width (n_bits): Specifies the width of the real/imaginary components.
      | Assumed equal for both components.
      | 
      | Binary Point (bin_pt): Specifies the binary point location in the real/imaginary components.
      | Assumed equal for both components.
      | </pre>
  requant{0..3} (4 alike) : xbsIndex_r3/Convert  arith_type="Signed  (2's comp)"  n_bits=9  bin_pt=0  quantization=Truncate  overflow=Wrap  latency=0  explicit_period=off  period=1  dbl_ovrd=off  show_param=on  inserted_by_tool=off  pipeline=on
      settings: xl_area=[0, 0, 0, 0, 0, 0, 0]
  ri_to_c : Subsystem
      mask Type: Real-Imag to Complex
      mask Description: Concatenates real and imaginary inputs into a complex output.
      mask Help:
      | <pre>
      | Description::
      | 
      | Concatenates a real and imaginary input into a complex output.
      | Useful for simplifying interconnects.
      | See also: Complex to Real-Imag (c_to_ri)
      | 
      | Mask Parameters::
      | 
      | (N/A)
      | </pre>
  ri_to_c1 : Subsystem
      mask Type: Real-Imag to Complex
      mask Description: Concatenates real and imaginary inputs into a complex output.
      mask Help:
      | <pre>
      | Description::
      | 
      | Concatenates a real and imaginary input into a complex output.
      | Useful for simplifying interconnects.
      | See also: Complex to Real-Imag (c_to_ri)
      | 
      | Mask Parameters::
      | 
      | (N/A)
      | </pre>
  shift{0..3} (4 alike) : xbsIndex_r3/Scale  scale_factor=0  explicit_period=off  period=1  dbl_ovrd=off
  sub_im : xbsIndex_r3/AddSub  mode=Subtraction  precision=Full  arith_type=Unsigned  n_bits=8  bin_pt=2  quantization=Truncate  overflow=Wrap  latency=1  explicit_period=off  period=1  use_carryin=off  use_carryout=off  en=off  dbl_ovrd=off  show_param=on  use_core=on  pipeline=on  use_rpm=on  gen_core=off
      settings: xl_area=[0, 0, 0, 0, 0, 0, 0]
  sub_re : xbsIndex_r3/AddSub  mode=Subtraction  precision=Full  arith_type=Unsigned  n_bits=8  bin_pt=2  quantization=Truncate  overflow=Wrap  latency=1  explicit_period=off  period=1  use_carryin=off  use_carryout=off  en=off  dbl_ovrd=off  show_param=on  use_core=on  pipeline=on  use_rpm=on  gen_core=off
      settings: xl_area=[0, 0, 0, 0, 0, 0, 0]
  a+b : Outport
  a-b : Outport  Port=2
  sync_out : Outport  Port=3
  wires:
  shift3/1 -> requant3/1
  sub_im/1 -> shift3/1
  shift2/1 -> requant2/1
  sub_re/1 -> shift2/1
  shift1/1 -> requant1/1
  shift0/1 -> requant0/1
  requant3/1 -> ri_to_c1/2(im)
  requant2/1 -> ri_to_c1/1(re)
  requant1/1 -> ri_to_c/2(im)
  requant0/1 -> ri_to_c/1(re)
  Delay/1 -> sync_out/1
  sync_in/1 -> Delay/1
  ri_to_c1/1(c) -> a-b/1
  ri_to_c/1(c) -> a+b/1
  add_im/1 -> shift1/1
  add_re/1 -> shift0/1
  a/1 -> c_to_ri/1(c)
  c_to_ri/2(im) -> sub_im/1, add_im/1
  c_to_ri/1(re) -> sub_re/1, add_re/1
  c_to_ri1/2(im) -> add_im/2, sub_im/2
  c_to_ri1/1(re) -> add_re/2, sub_re/2
  b/1 -> c_to_ri1/1(c)

== system test_newfft/r2_dit_fft/r2_dit_stage_1/r2_twiddle ==
  a_in : Inport  Port=1  LatchInput=off
  b_in : Inport  Port=2  LatchInput=off
  sync_in : Inport  Port=3  LatchInput=off
  a_out : Outport
  b_out : Outport  Port=2
  sync_out : Outport  Port=3
  wires:
  sync_in/1 -> sync_out/1
  b_in/1 -> b_out/1
  a_in/1 -> a_out/1

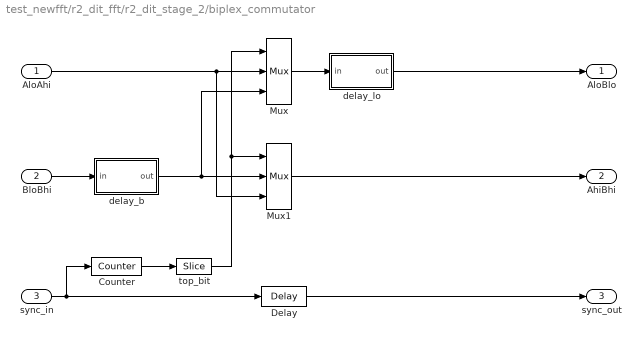
== system test_newfft/r2_dit_fft/r2_dit_stage_2/biplex_commutator ==
  AloAhi : Inport  Port=1  LatchInput=off
  BloBhi : Inport  Port=2  LatchInput=off
  sync_in : Inport  Port=3  LatchInput=off
  Counter : xbsIndex_r3/Counter  cnt_type=Free Running  n_bits=3  bin_pt=0  arith_type=Unsigned  start_count=0  cnt_to=Inf  cnt_by_val=1  operation=Up  explicit_period=off  period=1  load_pin=off  rst=on  en=off  dbl_ovrd=off  show_param=off  use_rpm=on  gen_core=off
      settings: xl_area=[0, 0, 0, 0, 0, 0, 0]
  Delay : xbsIndex_r3/Delay  latency=5  reg_retiming=off  explicit_period=off  period=1  en=off  accept_only_valid=off  init_zero=on  dbl_ovrd=off  show_param=off
      settings: xl_area=[0, 0, 0, 0, 0, 0, 0]
  Mux : xbsIndex_r3/Mux  inputs=2  precision=Full  arith_type="Signed  (2's comp)"  n_bits=8  bin_pt=2  quantization=Truncate  overflow=Wrap  latency=1  explicit_period=off  period=1  en=off  dbl_ovrd=off  show_param=off  mux_type=off  use_rpm=off  gen_core=off
      settings: xl_area=[0, 0, 0, 0, 0, 0, 0]
  Mux1 : xbsIndex_r3/Mux  inputs=2  precision=Full  arith_type="Signed  (2's comp)"  n_bits=8  bin_pt=2  quantization=Truncate  overflow=Wrap  latency=1  explicit_period=off  period=1  en=off  dbl_ovrd=off  show_param=on  mux_type=off  use_rpm=off  gen_core=off
      settings: xl_area=[0, 0, 0, 0, 0, 0, 0]
  delay_b : Subsystem  mask(SLR16 Delay){delay_depth=4}
      mask prompts: delay_depth "Delay Depth"
      mask help: A delay block that uses SLR16 elements for its storage.
      settings: AttributesFormatString=slr depth = 4
      mask Help:
      | <pre>
      | Description::
      | 
      | A delay block that uses SLR16 elements for its storage.
      | 
      | Mask Parameters::
      | 
      | Delay Depth (delay_depth): The length of the delay.
      | </pre>
  delay_lo : Subsystem  mask(SLR16 Delay){delay_depth=4}
      mask prompts: delay_depth "Delay Depth"
      mask help: A delay block that uses SLR16 elements for its storage.
      settings: AttributesFormatString=slr depth = 4
      mask Help:
      | <pre>
      | Description::
      | 
      | A delay block that uses SLR16 elements for its storage.
      | 
      | Mask Parameters::
      | 
      | Delay Depth (delay_depth): The length of the delay.
      | </pre>
  top_bit : xbsIndex_r3/Slice  mode=Upper Bit Location + Width  nbits=1  bit1=0  base1=MSB of Input  bit0=0  base0=LSB of Input  boolean_output=off  explicit_period=off  period=1  dbl_ovrd=off
  AloBlo : Outport
  AhiBhi : Outport  Port=2
  sync_out : Outport  Port=3
  wires:
  Delay/1 -> sync_out/1
  delay_lo/1(out) -> AloBlo/1
  Mux/1 -> delay_lo/1(in)
  delay_b/1(out) -> Mux/3, Mux1/2
  BloBhi/1 -> delay_b/1(in)
  Mux1/1 -> AhiBhi/1
  AloAhi/1 -> Mux1/3, Mux/2
  top_bit/1 -> Mux/1, Mux1/1
  Counter/1 -> top_bit/1
  sync_in/1 -> Delay/1, Counter/1

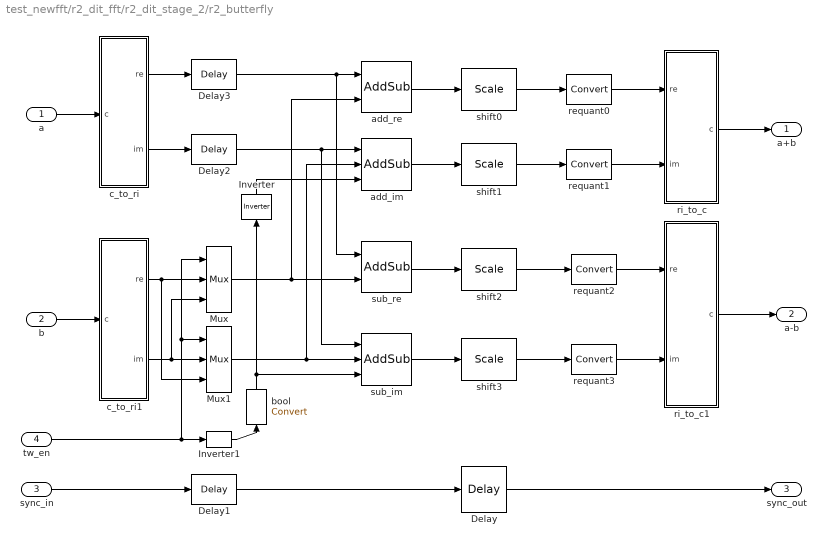
== system test_newfft/r2_dit_fft/r2_dit_stage_2/r2_butterfly ==
  a : Inport  Port=1  LatchInput=off
  b : Inport  Port=2  LatchInput=off
  sync_in : Inport  Port=3  LatchInput=off
  tw_en : Inport  Port=4  LatchInput=off
  Delay{,1..3} (4 alike) : xbsIndex_r3/Delay  latency=1  reg_retiming=off  explicit_period=off  period=1  en=off  accept_only_valid=off  init_zero=on  dbl_ovrd=off  show_param=off
      settings: xl_area=[0, 0, 0, 0, 0, 0, 0]
  Inverter : xbsIndex_r3/Inverter  Orientation=up  latency=0  explicit_period=off  period=1  en=off  dbl_ovrd=off  show_param=off
      settings: xl_area=[0, 0, 0, 0, 0, 0, 0]
  Inverter1 : xbsIndex_r3/Inverter  latency=1  explicit_period=off  period=1  en=off  dbl_ovrd=off  show_param=off
      settings: xl_area=[0, 0, 0, 0, 0, 0, 0]
  Mux : xbsIndex_r3/Mux  inputs=2  precision=Full  arith_type="Signed  (2's comp)"  n_bits=8  bin_pt=2  quantization=Truncate  overflow=Wrap  latency=1  explicit_period=off  period=1  en=off  dbl_ovrd=off  show_param=off  mux_type=off  use_rpm=off  gen_core=off
      settings: xl_area=[0, 0, 0, 0, 0, 0, 0]
  Mux1 : xbsIndex_r3/Mux  inputs=2  precision=Full  arith_type="Signed  (2's comp)"  n_bits=8  bin_pt=2  quantization=Truncate  overflow=Wrap  latency=1  explicit_period=off  period=1  en=off  dbl_ovrd=off  show_param=off  mux_type=off  use_rpm=off  gen_core=off
      settings: xl_area=[0, 0, 0, 0, 0, 0, 0]
  add_im : xbsIndex_r3/AddSub  mode=Addition or Subtraction  precision=Full  arith_type=Unsigned  n_bits=8  bin_pt=2  quantization=Truncate  overflow=Wrap  latency=1  explicit_period=off  period=1  use_carryin=off  use_carryout=off  en=off  dbl_ovrd=off  show_param=on  use_core=on  pipeline=on  use_rpm=on  gen_core=off
      settings: xl_area=[0, 0, 0, 0, 0, 0, 0]
  add_re : xbsIndex_r3/AddSub  mode=Addition  precision=Full  arith_type=Unsigned  n_bits=8  bin_pt=2  quantization=Truncate  overflow=Wrap  latency=1  explicit_period=off  period=1  use_carryin=off  use_carryout=off  en=off  dbl_ovrd=off  show_param=on  use_core=on  pipeline=on  use_rpm=on  gen_core=off
      settings: xl_area=[0, 0, 0, 0, 0, 0, 0]
  bool : xbsIndex_r3/Convert  Orientation=up  arith_type=Boolean  n_bits=8  bin_pt=6  quantization=Truncate  overflow=Wrap  latency=0  explicit_period=off  period=1  dbl_ovrd=off  show_param=off  inserted_by_tool=off  pipeline=off
      settings: xl_area=[0, 0, 0, 0, 0, 0, 0]
  c_to_ri : Subsystem  mask(Complex to Real-Imag){n_bits=9, bin_pt=0}
      mask prompts: n_bits "Bit Width"; bin_pt "Binary Point"
      mask help: Outputs real and imaginary components of a complex input.
      settings: AttributesFormatString=9_0 r/i
      mask Help:
      | <pre>
      | Description::
      | 
      | Outputs real and imaginary components of a complex input.
      | Useful for simplifying interconnects.
      | See also: Real-Imag to Complex (ri_to_c)
      | 
      | Mask Parameters::
      | 
      | Bit Width (n_bits): Specifies the width of the real/imaginary components.
      | Assumed equal for both components.
      | 
      | Binary Point (bin_pt): Specifies the binary point location in the real/imaginary components.
      | Assumed equal for both components.
      | </pre>
  c_to_ri1 : Subsystem  mask(Complex to Real-Imag){n_bits=9, bin_pt=0}
      mask prompts: n_bits "Bit Width"; bin_pt "Binary Point"
      mask help: Outputs real and imaginary components of a complex input.
      settings: AttributesFormatString=9_0 r/i
      mask Help:
      | <pre>
      | Description::
      | 
      | Outputs real and imaginary components of a complex input.
      | Useful for simplifying interconnects.
      | See also: Real-Imag to Complex (ri_to_c)
      | 
      | Mask Parameters::
      | 
      | Bit Width (n_bits): Specifies the width of the real/imaginary components.
      | Assumed equal for both components.
      | 
      | Binary Point (bin_pt): Specifies the binary point location in the real/imaginary components.
      | Assumed equal for both components.
      | </pre>
  requant{0..3} (4 alike) : xbsIndex_r3/Convert  arith_type="Signed  (2's comp)"  n_bits=10  bin_pt=0  quantization=Truncate  overflow=Wrap  latency=0  explicit_period=off  period=1  dbl_ovrd=off  show_param=on  inserted_by_tool=off  pipeline=on
      settings: xl_area=[0, 0, 0, 0, 0, 0, 0]
  ri_to_c : Subsystem
      mask Type: Real-Imag to Complex
      mask Description: Concatenates real and imaginary inputs into a complex output.
      mask Help:
      | <pre>
      | Description::
      | 
      | Concatenates a real and imaginary input into a complex output.
      | Useful for simplifying interconnects.
      | See also: Complex to Real-Imag (c_to_ri)
      | 
      | Mask Parameters::
      | 
      | (N/A)
      | </pre>
  ri_to_c1 : Subsystem
      mask Type: Real-Imag to Complex
      mask Description: Concatenates real and imaginary inputs into a complex output.
      mask Help:
      | <pre>
      | Description::
      | 
      | Concatenates a real and imaginary input into a complex output.
      | Useful for simplifying interconnects.
      | See also: Complex to Real-Imag (c_to_ri)
      | 
      | Mask Parameters::
      | 
      | (N/A)
      | </pre>
  shift{0..3} (4 alike) : xbsIndex_r3/Scale  scale_factor=0  explicit_period=off  period=1  dbl_ovrd=off
  sub_im : xbsIndex_r3/AddSub  mode=Addition or Subtraction  precision=Full  arith_type=Unsigned  n_bits=8  bin_pt=2  quantization=Truncate  overflow=Wrap  latency=1  explicit_period=off  period=1  use_carryin=off  use_carryout=off  en=off  dbl_ovrd=off  show_param=on  use_core=on  pipeline=on  use_rpm=on  gen_core=off
      settings: xl_area=[0, 0, 0, 0, 0, 0, 0]
  sub_re : xbsIndex_r3/AddSub  mode=Subtraction  precision=Full  arith_type=Unsigned  n_bits=8  bin_pt=2  quantization=Truncate  overflow=Wrap  latency=1  explicit_period=off  period=1  use_carryin=off  use_carryout=off  en=off  dbl_ovrd=off  show_param=on  use_core=on  pipeline=on  use_rpm=on  gen_core=off
      settings: xl_area=[0, 0, 0, 0, 0, 0, 0]
  a+b : Outport
  a-b : Outport  Port=2
  sync_out : Outport  Port=3
  wires:
  add_im/1 -> shift1/1
  sub_im/1 -> shift3/1
  sub_re/1 -> shift2/1
  requant3/1 -> ri_to_c1/2(im)
  requant2/1 -> ri_to_c1/1(re)
  requant1/1 -> ri_to_c/2(im)
  requant0/1 -> ri_to_c/1(re)
  add_re/1 -> shift0/1
  shift3/1 -> requant3/1
  shift2/1 -> requant2/1
  shift1/1 -> requant1/1
  shift0/1 -> requant0/1
  bool/1 -> Inverter/1, sub_im/3
  Inverter/1 -> add_im/3
  Inverter1/1 -> bool/1
  Mux/1 -> sub_re/2, add_re/2
  Delay3/1 -> add_re/1, sub_re/1
  Delay2/1 -> add_im/1, sub_im/1
  Mux1/1 -> add_im/2, sub_im/2
  Delay1/1 -> Delay/1
  tw_en/1 -> Inverter1/1, Mux1/1, Mux/1
  c_to_ri1/2(im) -> Mux/3, Mux1/2
  c_to_ri1/1(re) -> Mux1/3, Mux/2
  b/1 -> c_to_ri1/1(c)
  c_to_ri/1(re) -> Delay3/1
  c_to_ri/2(im) -> Delay2/1
  a/1 -> c_to_ri/1(c)
  ri_to_c/1(c) -> a+b/1
  ri_to_c1/1(c) -> a-b/1
  sync_in/1 -> Delay1/1
  Delay/1 -> sync_out/1

== system test_newfft/r2_dit_fft/r2_dit_stage_2/r2_twiddle ==
  a_in : Inport  Port=1  LatchInput=off
  b_in : Inport  Port=2  LatchInput=off
  sync_in : Inport  Port=3  LatchInput=off
  Counter : xbsIndex_r3/Counter  cnt_type=Free Running  n_bits=3  bin_pt=0  arith_type=Unsigned  start_count=0  cnt_to=Inf  cnt_by_val=1  operation=Up  explicit_period=off  period=1  load_pin=off  rst=on  en=off  dbl_ovrd=off  show_param=on  use_rpm=on  gen_core=off
      settings: xl_area=[0, 0, 0, 0, 0, 0, 0]
  top_bit : xbsIndex_r3/Slice  mode=Upper Bit Location + Width  nbits=1  bit1=0  base1=MSB of Input  bit0=0  base0=LSB of Input  boolean_output=off  explicit_period=off  period=1  dbl_ovrd=off
  a_out : Outport
  b_out : Outport  Port=2
  sync_out : Outport  Port=3
  tw_en : Outport  Port=4
  wires:
  b_in/1 -> b_out/1
  a_in/1 -> a_out/1
  top_bit/1 -> tw_en/1
  Counter/1 -> top_bit/1
  sync_in/1 -> sync_out/1, Counter/1
